simulink model "RequirementsTable"  (R2022a)
settings: Solver=VariableStepAuto  StartTime=0.0  StopTime=10.0  RelTol=1e-3
undefined symbols (not defined in the file): ATR_PULSE_WIDTH, ATR_RP, HEART_RATE, VENT_PULSE_WIDTH, VENT_RP
settings Model: Creator=aldra  LastModifiedBy=bkfre
settings ModelReferenceCC: EnableRefExpFcnMdlSchedulingChecks=off
settings RTWCC: Description=Generic Real-Time Target

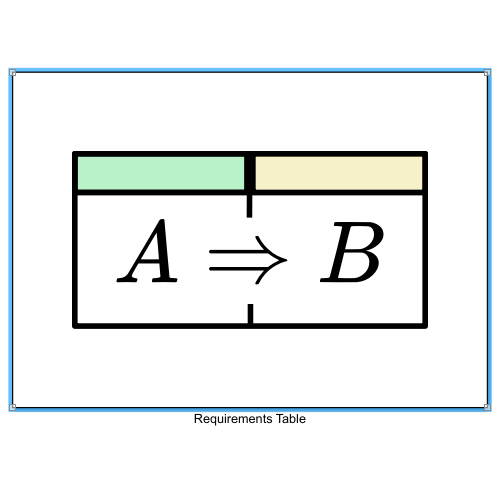
[thumbnail: Simulink's stored preview of the top-level diagram]
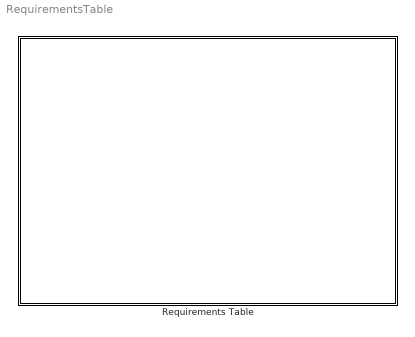
== system RequirementsTable ==
  Requirements Table : Requirements Table  TreatAsAtomicUnit=on

== stateflow chart RequirementsTable/Requirements Table ==
  (default) -> (junction 1073742835)
  (junction 1073742835) -> (junction 1073742836) : {
      | % SF_REQ_REV_07
      | }
  (junction 1073742836) -> (junction 1073742838) : {
      | % HEADER_ASSIGNMENTS
      |
      | }
  (junction 1073742838) -> (junction 1073742840) : {
      | % START_A_4
      | }
  (junction 1073742840) -> (junction 1073742842) : {
      | }
  (junction 1073742842) -> (junction 1073742844)
  (junction 1073742844) -> (junction 1073742846) : {
      | }
  (junction 1073742846) -> (junction 1073742848) : {
      | % END_A_4
      | }
  (junction 1073742848) -> (junction 1073743264) : {
      | % START_R_64
      | }
  (junction 1073743264) -> (junction 1073743266) : {
      | }
  (junction 1073743266) -> (junction 1073743268) : {
      |
      |
      | }
  (junction 1073743268) -> (junction 1073743270) : {
      | }
  (junction 1073743270) -> (junction 1073743338) : {
      | % START_R_70
      | }
  (junction 1073743338) -> (junction 1073743340) : {
      | }
  (junction 1073743340) -> (junction 1073743342)
  (junction 1073743342) -> (junction 1073743344) [order 1] : [(((MODE) == (AOO or VOO or AAI or VVI)))]
  (junction 1073743342) -> (junction 1073743350) [order 2]
  (junction 1073743344) -> (junction 1073743346) : {
      | HEART_RATE = LRL
      |
      | }
  (junction 1073743346) -> (junction 1073743348) : {
      | }
  (junction 1073743348) -> (junction 1073743350)
  (junction 1073743350) -> (junction 1073743352)
  (junction 1073743352) -> (junction 1073743354) : {
      | % END_R_70
      | }
  (junction 1073743354) -> (junction 1073743371) : {
      | % START_R_73
      | }
  (junction 1073743371) -> (junction 1073743373) : {
      | }
  (junction 1073743373) -> (junction 1073743375)
  (junction 1073743375) -> (junction 1073743377) [order 1] : [(((MODE) == (AOOR or VOOR or AAIR or VVIR)))]
  (junction 1073743375) -> (junction 1073743383) [order 2]
  (junction 1073743377) -> (junction 1073743379) : {
      | HEART_RATE = RATE_MOD
      |
      | }
  (junction 1073743379) -> (junction 1073743381) : {
      | }
  (junction 1073743381) -> (junction 1073743383)
  (junction 1073743383) -> (junction 1073743385)
  (junction 1073743385) -> (junction 1073743387) : {
      | % END_R_73
      | }
  (junction 1073743387) -> (junction 1073743404) : {
      | % START_R_76
      | }
  (junction 1073743404) -> (junction 1073743406) : {
      | }
  (junction 1073743406) -> (junction 1073743408)
  (junction 1073743408) -> (junction 1073743410) [order 1] : [(((INPUT) == (HEART_RATE < LRL)))]
  (junction 1073743408) -> (junction 1073743416) [order 2]
  (junction 1073743410) -> (junction 1073743412) : {
      | HEART_RATE = LRL
      |
      | }
  (junction 1073743412) -> (junction 1073743414) : {
      | }
  (junction 1073743414) -> (junction 1073743416)
  (junction 1073743416) -> (junction 1073743418)
  (junction 1073743418) -> (junction 1073743420) : {
      | % END_R_76
      | }
  (junction 1073743420) -> (junction 1073743437) : {
      | % START_R_79
      | }
  (junction 1073743437) -> (junction 1073743439) : {
      | }
  (junction 1073743439) -> (junction 1073743441)
  (junction 1073743441) -> (junction 1073743443) [order 1] : [(((INPUT) == (HEART_RATE > URL)))]
  (junction 1073743441) -> (junction 1073743449) [order 2]
  (junction 1073743443) -> (junction 1073743445) : {
      | HEART_RATE = URL
      |
      | }
  (junction 1073743445) -> (junction 1073743447) : {
      | }
  (junction 1073743447) -> (junction 1073743449)
  (junction 1073743449) -> (junction 1073743451)
  (junction 1073743451) -> (junction 1073743453) : {
      | % END_R_79
      | }
  (junction 1073743453) -> (junction 1073743282) : {
      | % END_R_64
      | }
  (junction 1073743282) -> (junction 1073742850) : {
      | % START_R_1
      | }
  (junction 1073742850) -> (junction 1073742852) : {
      | }
  (junction 1073742852) -> (junction 1073742854)
  (junction 1073742854) -> (junction 1073742856) [order 1] : [(((MODE) == (AOO or AOOR)))]
  (junction 1073742854) -> (junction 1073742898) [order 2]
  (junction 1073742856) -> (junction 1073742858) : {
      |
      |
      | }
  (junction 1073742858) -> (junction 1073742860) : {
      | }
  (junction 1073742860) -> (junction 1073742862) : {
      | % START_R_13
      | }
  (junction 1073742862) -> (junction 1073742864) : {
      | }
  (junction 1073742864) -> (junction 1073742866)
  (junction 1073742866) -> (junction 1073742868) [order 1] : [duration((((STATE) == (IDLE)))) >= 60000/HEART_RATE]
  (junction 1073742866) -> (junction 1073742874) [order 2]
  (junction 1073742868) -> (junction 1073742870) : {
      | PACE_ATRIUM
      |
      | }
  (junction 1073742870) -> (junction 1073742872) : {
      | }
  (junction 1073742872) -> (junction 1073742874)
  (junction 1073742874) -> (junction 1073742876)
  (junction 1073742876) -> (junction 1073742878) : {
      | % END_R_13
      | }
  (junction 1073742878) -> (junction 1073742880) : {
      | % START_R_16
      | }
  (junction 1073742880) -> (junction 1073742882) : {
      | }
  (junction 1073742882) -> (junction 1073742884)
  (junction 1073742884) -> (junction 1073742886) [order 1] : [duration((((STATE) == (PACE_ATRIUM)))) >= ATR_PULSE_WIDTH]
  (junction 1073742884) -> (junction 1073742892) [order 2]
  (junction 1073742886) -> (junction 1073742888) : {
      | IDLE
      |
      | }
  (junction 1073742888) -> (junction 1073742890) : {
      | }
  (junction 1073742890) -> (junction 1073742892)
  (junction 1073742892) -> (junction 1073742894)
  (junction 1073742894) -> (junction 1073742896) : {
      | % END_R_16
      | }
  (junction 1073742896) -> (junction 1073742898)
  (junction 1073742898) -> (junction 1073742900)
  (junction 1073742900) -> (junction 1073743236) : {
      | % END_R_1
      | }
  (junction 1073743236) -> (junction 1073742904) : {
      | % START_R_10
      | }
  (junction 1073742904) -> (junction 1073742906) : {
      | }
  (junction 1073742906) -> (junction 1073742908)
  (junction 1073742908) -> (junction 1073742910) [order 1] : [(((MODE) == (AAI or AAIR)))]
  (junction 1073742908) -> (junction 1073742970) [order 2]
  (junction 1073742910) -> (junction 1073742912) : {
      |
      |
      | }
  (junction 1073742912) -> (junction 1073742914) : {
      | }
  (junction 1073742914) -> (junction 1073742916) : {
      | % START_R_22
      | }
  (junction 1073742916) -> (junction 1073742918) : {
      | }
  (junction 1073742918) -> (junction 1073742920)
  (junction 1073742920) -> (junction 1073742922) [order 1] : [duration((((STATE) == (REFRACTORY)))) >= ATR_RP]
  (junction 1073742920) -> (junction 1073742928) [order 2]
  (junction 1073742922) -> (junction 1073742924) : {
      | ALERT
      |
      | }
  (junction 1073742924) -> (junction 1073742926) : {
      | }
  (junction 1073742926) -> (junction 1073742928)
  (junction 1073742928) -> (junction 1073742930)
  (junction 1073742930) -> (junction 1073742932) : {
      | % END_R_22
      | }
  (junction 1073742932) -> (junction 1073742934) : {
      | % START_R_25
      | }
  (junction 1073742934) -> (junction 1073742936) : {
      | }
  (junction 1073742936) -> (junction 1073742938)
  (junction 1073742938) -> (junction 1073742940) [order 1] : [(((STATE) == (ALERT)))]
  (junction 1073742938) -> (junction 1073742964) [order 2]
  (junction 1073742940) -> (junction 1073742942) : {
      |
      |
      | }
  (junction 1073742942) -> (junction 1073742944) : {
      | }
  (junction 1073742944) -> (junction 1073742946) : {
      | % START_R_28
      | }
  (junction 1073742946) -> (junction 1073742948) : {
      | }
  (junction 1073742948) -> (junction 1073742950)
  (junction 1073742950) -> (junction 1073742952) [order 1] : [duration((((INPUT) == (P_WAVE==1)))) >= 0]
  (junction 1073742950) -> (junction 1073742958) [order 2]
  (junction 1073742952) -> (junction 1073742954) : {
      | REFRACTORY
      |
      | }
  (junction 1073742954) -> (junction 1073742956) : {
      | }
  (junction 1073742956) -> (junction 1073742958)
  (junction 1073742958) -> (junction 1073742960)
  (junction 1073742960) -> (junction 1073742962) : {
      | % END_R_28
      | }
  (junction 1073742962) -> (junction 1073742997) : {
      | % START_R_31
      | }
  (junction 1073742997) -> (junction 1073742999) : {
      | }
  (junction 1073742999) -> (junction 1073743001)
  (junction 1073743001) -> (junction 1073743003) [order 1] : [duration((((INPUT) == (P_WAVE==0)))) >= 60000/HEART_RATE - ATR_RP]
  (junction 1073743001) -> (junction 1073743009) [order 2]
  (junction 1073743003) -> (junction 1073743005) : {
      | PACE_ATRIUM
      |
      | }
  (junction 1073743005) -> (junction 1073743007) : {
      | }
  (junction 1073743007) -> (junction 1073743009)
  (junction 1073743009) -> (junction 1073743011)
  (junction 1073743011) -> (junction 1073743013) : {
      | % END_R_31
      | }
  (junction 1073743013) -> (junction 1073742964)
  (junction 1073742964) -> (junction 1073742966)
  (junction 1073742966) -> (junction 1073742968) : {
      | % END_R_25
      | }
  (junction 1073742968) -> (junction 1073743030) : {
      | % START_R_34
      | }
  (junction 1073743030) -> (junction 1073743032) : {
      | }
  (junction 1073743032) -> (junction 1073743034)
  (junction 1073743034) -> (junction 1073743036) [order 1] : [duration((((STATE) == (PACE_ATRIUM)))) >= ATR_PULSE_WIDTH]
  (junction 1073743034) -> (junction 1073743042) [order 2]
  (junction 1073743036) -> (junction 1073743038) : {
      | REFRACTORY
      |
      | }
  (junction 1073743038) -> (junction 1073743040) : {
      | }
  (junction 1073743040) -> (junction 1073743042)
  (junction 1073743042) -> (junction 1073743044)
  (junction 1073743044) -> (junction 1073743046) : {
      | % END_R_34
      | }
  (junction 1073743046) -> (junction 1073742970)
  (junction 1073742970) -> (junction 1073742972)
  (junction 1073742972) -> (junction 1073742974) : {
      | % END_R_10
      | }
  (junction 1073742974) -> (junction 1073743052) : {
      | % START_R_37
      | }
  (junction 1073743052) -> (junction 1073743054) : {
      | }
  (junction 1073743054) -> (junction 1073743056)
  (junction 1073743056) -> (junction 1073743058) [order 1] : [(((MODE) == (VOO or VOOR)))]
  (junction 1073743056) -> (junction 1073743100) [order 2]
  (junction 1073743058) -> (junction 1073743060) : {
      |
      |
      | }
  (junction 1073743060) -> (junction 1073743062) : {
      | }
  (junction 1073743062) -> (junction 1073743064) : {
      | % START_R_40
      | }
  (junction 1073743064) -> (junction 1073743066) : {
      | }
  (junction 1073743066) -> (junction 1073743068)
  (junction 1073743068) -> (junction 1073743070) [order 1] : [duration((((STATE) == (IDLE)))) >= 60000/HEART_RATE]
  (junction 1073743068) -> (junction 1073743076) [order 2]
  (junction 1073743070) -> (junction 1073743072) : {
      | PACE_VENTRICLE
      |
      | }
  (junction 1073743072) -> (junction 1073743074) : {
      | }
  (junction 1073743074) -> (junction 1073743076)
  (junction 1073743076) -> (junction 1073743078)
  (junction 1073743078) -> (junction 1073743080) : {
      | % END_R_40
      | }
  (junction 1073743080) -> (junction 1073743082) : {
      | % START_R_43
      | }
  (junction 1073743082) -> (junction 1073743084) : {
      | }
  (junction 1073743084) -> (junction 1073743086)
  (junction 1073743086) -> (junction 1073743088) [order 1] : [duration((((STATE) == (PACE_VENTRICLE)))) >= VENT_PULSE_WIDTH]
  (junction 1073743086) -> (junction 1073743094) [order 2]
  (junction 1073743088) -> (junction 1073743090) : {
      | IDLE
      |
      | }
  (junction 1073743090) -> (junction 1073743092) : {
      | }
  (junction 1073743092) -> (junction 1073743094)
  (junction 1073743094) -> (junction 1073743096)
  (junction 1073743096) -> (junction 1073743098) : {
      | % END_R_43
      | }
  (junction 1073743098) -> (junction 1073743100)
  (junction 1073743100) -> (junction 1073743102)
  (junction 1073743102) -> (junction 1073743104) : {
      | % END_R_37
      | }
  (junction 1073743104) -> (junction 1073743106) : {
      | % START_R_46
      | }
  (junction 1073743106) -> (junction 1073743108) : {
      | }
  (junction 1073743108) -> (junction 1073743110)
  (junction 1073743110) -> (junction 1073743112) [order 1] : [(((MODE) == (VVI or VVIR)))]
  (junction 1073743110) -> (junction 1073743208) [order 2]
  (junction 1073743112) -> (junction 1073743114) : {
      |
      |
      | }
  (junction 1073743114) -> (junction 1073743116) : {
      | }
  (junction 1073743116) -> (junction 1073743118) : {
      | % START_R_49
      | }
  (junction 1073743118) -> (junction 1073743120) : {
      | }
  (junction 1073743120) -> (junction 1073743122)
  (junction 1073743122) -> (junction 1073743124) [order 1] : [duration((((STATE) == (REFRACTORY)))) >= VENT_RP]
  (junction 1073743122) -> (junction 1073743130) [order 2]
  (junction 1073743124) -> (junction 1073743126) : {
      | ALERT
      |
      | }
  (junction 1073743126) -> (junction 1073743128) : {
      | }
  (junction 1073743128) -> (junction 1073743130)
  (junction 1073743130) -> (junction 1073743132)
  (junction 1073743132) -> (junction 1073743134) : {
      | % END_R_49
      | }
  (junction 1073743134) -> (junction 1073743136) : {
      | % START_R_52
      | }
  (junction 1073743136) -> (junction 1073743138) : {
      | }
  (junction 1073743138) -> (junction 1073743140)
  (junction 1073743140) -> (junction 1073743142) [order 1] : [(((STATE) == (ALERT)))]
  (junction 1073743140) -> (junction 1073743184) [order 2]
  (junction 1073743142) -> (junction 1073743144) : {
      |
      |
      | }
  (junction 1073743144) -> (junction 1073743146) : {
      | }
  (junction 1073743146) -> (junction 1073743148) : {
      | % START_R_55
      | }
  (junction 1073743148) -> (junction 1073743150) : {
      | }
  (junction 1073743150) -> (junction 1073743152)
  (junction 1073743152) -> (junction 1073743154) [order 1] : [duration((((INPUT) == (R_WAVE==1)))) >= 0]
  (junction 1073743152) -> (junction 1073743160) [order 2]
  (junction 1073743154) -> (junction 1073743156) : {
      | REFRACTORY
      |
      | }
  (junction 1073743156) -> (junction 1073743158) : {
      | }
  (junction 1073743158) -> (junction 1073743160)
  (junction 1073743160) -> (junction 1073743162)
  (junction 1073743162) -> (junction 1073743164) : {
      | % END_R_55
      | }
  (junction 1073743164) -> (junction 1073743166) : {
      | % START_R_58
      | }
  (junction 1073743166) -> (junction 1073743168) : {
      | }
  (junction 1073743168) -> (junction 1073743170)
  (junction 1073743170) -> (junction 1073743172) [order 1] : [duration((((INPUT) == (R_WAVE==0)))) >= 60000/HEART_RATE - VENT_RP]
  (junction 1073743170) -> (junction 1073743178) [order 2]
  (junction 1073743172) -> (junction 1073743174) : {
      | PACE_VENTRICLE
      |
      | }
  (junction 1073743174) -> (junction 1073743176) : {
      | }
  (junction 1073743176) -> (junction 1073743178)
  (junction 1073743178) -> (junction 1073743180)
  (junction 1073743180) -> (junction 1073743182) : {
      | % END_R_58
      | }
  (junction 1073743182) -> (junction 1073743184)
  (junction 1073743184) -> (junction 1073743186)
  (junction 1073743186) -> (junction 1073743188) : {
      | % END_R_52
      | }
  (junction 1073743188) -> (junction 1073743190) : {
      | % START_R_61
      | }
  (junction 1073743190) -> (junction 1073743192) : {
      | }
  (junction 1073743192) -> (junction 1073743194)
  (junction 1073743194) -> (junction 1073743196) [order 1] : [duration((((STATE) == (PACE_VENTRICLE)))) >= VENT_PULSE_WIDTH]
  (junction 1073743194) -> (junction 1073743202) [order 2]
  (junction 1073743196) -> (junction 1073743198) : {
      | REFRACTORY
      |
      | }
  (junction 1073743198) -> (junction 1073743200) : {
      | }
  (junction 1073743200) -> (junction 1073743202)
  (junction 1073743202) -> (junction 1073743204)
  (junction 1073743204) -> (junction 1073743206) : {
      | % END_R_61
      | }
  (junction 1073743206) -> (junction 1073743208)
  (junction 1073743208) -> (junction 1073743210)
  (junction 1073743210) -> (junction 1073743212) : {
      | % END_R_46
      | }
  data: HEART_RATE parameter; ATR_PULSE_WIDTH parameter; ATR_RP parameter; VENT_PULSE_WIDTH parameter; VENT_RP parameter
